simulink model "nlQuadtank"  (Simulink 10.3)
settings: Solver=ode4  StartTime=0.0  StopTime=50  FixedStep=0.001  RelTol=1e-3  EnableMultiTasking=on
values from neighbouring files (symbols this model uses):
  a1 = 0.071    [quadtank.m]    (also in quadtank_minphase.m; quadtank_nonminphase.m; symbolic_linearisation.m)
  A1 = 30    [quadtank.m]    (also in quadtank_minphase.m; quadtank_nonminphase.m; symbolic_linearisation.m)
  a2 = 0.057    [quadtank.m]    (also in quadtank_minphase.m; quadtank_nonminphase.m; symbolic_linearisation.m)
  A2 = 35    [quadtank.m]    (also in quadtank_minphase.m; quadtank_nonminphase.m; symbolic_linearisation.m)
  a3 = 0.071    [quadtank.m]    (also in quadtank_minphase.m; quadtank_nonminphase.m; symbolic_linearisation.m)
  A3 = 30    [quadtank.m]    (also in quadtank_minphase.m; quadtank_nonminphase.m; symbolic_linearisation.m)
  a4 = 0.057    [quadtank.m]    (also in quadtank_minphase.m; quadtank_nonminphase.m; symbolic_linearisation.m)
  A4 = 35    [quadtank.m]    (also in quadtank_minphase.m; quadtank_nonminphase.m; symbolic_linearisation.m)
  g = 981    [quadtank.m]    (also in quadtank_minphase.m; quadtank_nonminphase.m; symbolic_linearisation.m)
  g1 = par(mode).g1    [quadtank.m]    (also in quadtank_minphase.m = par(1).g1; quadtank_nonminphase.m = par(2).g1; symbolic_linearisation.m = par(2).g1)
  g2 = par(mode).g2    [quadtank.m]    (also in quadtank_minphase.m = par(1).g2; quadtank_nonminphase.m = par(2).g2; symbolic_linearisation.m = par(2).g2)
  h10 = par(mode).h10    [quadtank.m]    (also in quadtank_minphase.m = par(1).h10; quadtank_nonminphase.m = par(2).h10; symbolic_linearisation.m = par(2).h10)
  h20 = par(mode).h20    [quadtank.m]    (also in quadtank_minphase.m = par(1).h20; quadtank_nonminphase.m = par(2).h20; symbolic_linearisation.m = par(2).h20)
  h30 = par(mode).h30    [quadtank.m]    (also in quadtank_minphase.m = par(1).h30; quadtank_nonminphase.m = par(2).h30; symbolic_linearisation.m = par(2).h30)
  h40 = par(mode).h40    [quadtank.m]    (also in quadtank_minphase.m = par(1).h40; quadtank_nonminphase.m = par(2).h40; symbolic_linearisation.m = par(2).h40)
  k1 = par(mode).k1    [quadtank.m]    (also in quadtank_minphase.m = par(1).k1; quadtank_nonminphase.m = par(2).k1; symbolic_linearisation.m = par(2).k1)
  k2 = par(mode).k2    [quadtank.m]    (also in quadtank_minphase.m = par(1).k2; quadtank_nonminphase.m = par(2).k2; symbolic_linearisation.m = par(2).k2)
settings Model: Creator=misgeld  LastModifiedBy=mspms
settings DataIOCC: LimitDataPoints=on
settings DebuggingCC: UnderspecifiedInitializationDetection=Simplified  MergeDetectMultiDrivingBlocksExec=error  SolverPrmCheckMsg=warning

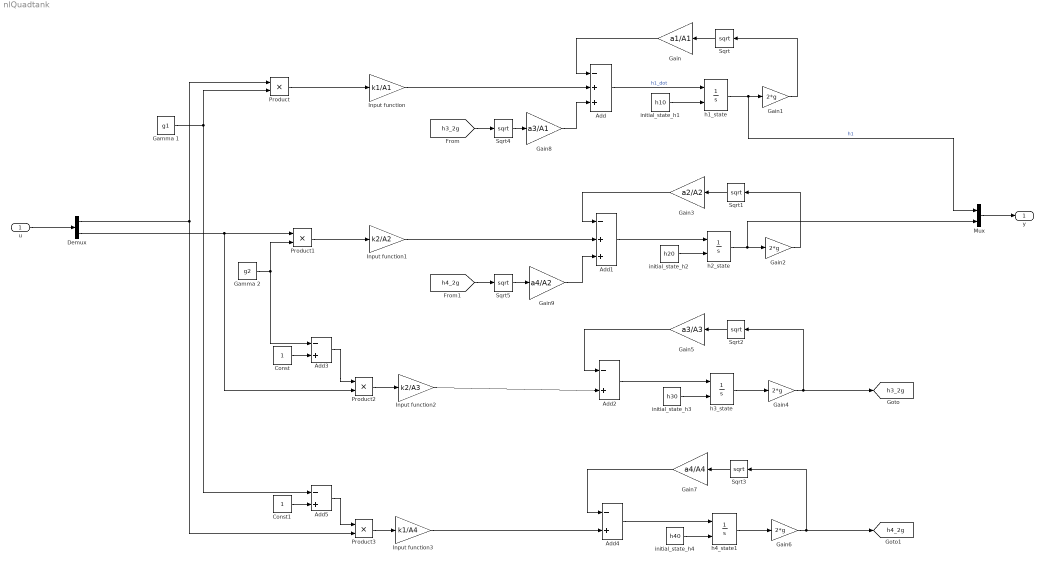
== system nlQuadtank ==
  u : Inport
  Add : Sum  Inputs=-++
  Add1 : Sum  Inputs=-++
  Add{2..5} (4 alike) : Sum  Inputs=-+
  Const : Constant
  Const1 : Constant
  Demux : Demux  Outputs=2
  Gain : Gain  Gain=a1/A1
  Gain{1..2,4,6} (4 alike) : Gain  Gain=2*g
  Gain3 : Gain  Gain=a2/A2
  Gain5 : Gain  Gain=a3/A3
  Gain7 : Gain  Gain=a4/A4
  Gain8 : Gain  Gain=a3/A1
  Gain9 : Gain  Gain=a4/A2
  Gamma 1 : Constant  Value=g1
  Gamma 2 : Constant  Value=g2
  Input function : Gain  Gain=k1/A1
  Input function1 : Gain  Gain=k2/A2
  Input function2 : Gain  Gain=k2/A3
  Input function3 : Gain  Gain=k1/A4
  Mux : Mux  Inputs=2
  Product{,1..3} (4 alike) : Product  RndMeth=Zero
  Sqrt{,1..5} (6 alike) : Sqrt  SaturateOnIntegerOverflow=on
  h1_state : Integrator  InitialConditionSource=external
  h2_state : Integrator  InitialConditionSource=external
  h3_state : Integrator  InitialConditionSource=external
  h4_state1 : Integrator  InitialConditionSource=external
  initial_state_h1 : Constant  Value=h10
  initial_state_h2 : Constant  Value=h20
  initial_state_h3 : Constant  Value=h30
  initial_state_h4 : Constant  Value=h40
  y : Outport
  tag scope: h3_2g=global, h4_2g=global
  wires:
  Demux/1 -> Product/1, Product3/2
  Product/1 -> Input function/1
  Gamma 1/1 -> Product/2, Add5/1
  Input function/1 -> Add/2
  Add/1 -> h1_state/1  "h1_dot"
  initial_state_h1/1 -> h1_state/2
  Sqrt/1 -> Gain/1
  h1_state/1 -> Gain1/1, Mux/1  "h1"
  Gain1/1 -> Sqrt/1
  Gain/1 -> Add/1
  Add1/1 -> h2_state/1
  initial_state_h2/1 -> h2_state/2
  h2_state/1 -> Mux/2, Gain2/1
  Gain2/1 -> Sqrt1/1
  Sqrt1/1 -> Gain3/1
  Gain3/1 -> Add1/1
  Demux/2 -> Product1/1, Product2/2
  Gamma 2/1 -> Product1/2, Add3/1
  Product1/1 -> Input function1/1
  Input function1/1 -> Add1/2
  Add2/1 -> h3_state/1
  initial_state_h3/1 -> h3_state/2
  h3_state/1 -> Gain4/1
  Input function2/1 -> Add2/2
  Product2/1 -> Input function2/1
  Const/1 -> Add3/2
  Add3/1 -> Product2/1
  Sqrt2/1 -> Gain5/1
  Gain4/1 -> Sqrt2/1, [h3_2g]
  Gain5/1 -> Add2/1
  Add4/1 -> h4_state1/1
  initial_state_h4/1 -> h4_state1/2
  h4_state1/1 -> Gain6/1
  Input function3/1 -> Add4/2
  Sqrt3/1 -> Gain7/1
  Gain6/1 -> Sqrt3/1, [h4_2g]
  Gain7/1 -> Add4/1
  Product3/1 -> Input function3/1
  Add5/1 -> Product3/1
  Const1/1 -> Add5/2
  Gain8/1 -> Add/3
  Sqrt4/1 -> Gain8/1
  [h3_2g] -> Sqrt4/1
  Gain9/1 -> Add1/3
  Sqrt5/1 -> Gain9/1
  [h4_2g] -> Sqrt5/1
  Mux/1 -> y/1
  u/1 -> Demux/1
